simulink model "A03_L5_2"  (R2018b)
settings: Solver=ode45  StartTime=0.0  StopTime=60  MaxStep=0.01  RelTol=1e-3  EnableMultiTasking=on
values from neighbouring files (symbols this model uses):
  K = 2    [A04_L5_script.m]
  T = 1.1+0.3*a+0.6*b    (= 3.5)    [A04_L5_script.m]
  y0 = 0    [A04_L5_script.m]
settings Model: Creator=User  LastModifiedBy=DRAGOMIR
settings DataIOCC: LimitDataPoints=on  SaveFormat=Array
settings OptimizationCC: LifeSpan=inf
settings DebuggingCC: SolverPrmCheckMsg=warning  SFUnexpectedBacktrackingDiag=warning  SFNoUnconditionalDefaultTransitionDiag=warning  SFExecutionAtInitializationDiag=none
settings HardwareCC: ProdBitPerPointer=32  ProdBitPerSizeT=32  ProdBitPerPtrDiffT=32  ProdLargestAtomicFloat=None  ProdIntDivRoundTo=Undefined  ProdEndianess=Unspecified  ProdWordSize=32  ProdHWDeviceType=32-bit Generic
settings ModelReferenceCC: PropagateSignalLabelsOutOfModel=off
settings SFSimCC: SimUseLocalCustomCode=off
settings RTWCC: RTWUseLocalCustomCode=off
settings CodeAppCC: StateflowObjectComments=on
settings GRTTargetCC: TargetLangStandard=C89/C90 (ANSI)  GeneratePreprocessorConditionals=Disable all
settings ConfigComp: CovMetricSettings=dw  CovHtmlReporting=on  CovSaveCumulativeToWorkspaceVar=on  CovSaveSingleToWorkspaceVar=on  CovExternalEMLEnable=off  CovSFcnEnable=off

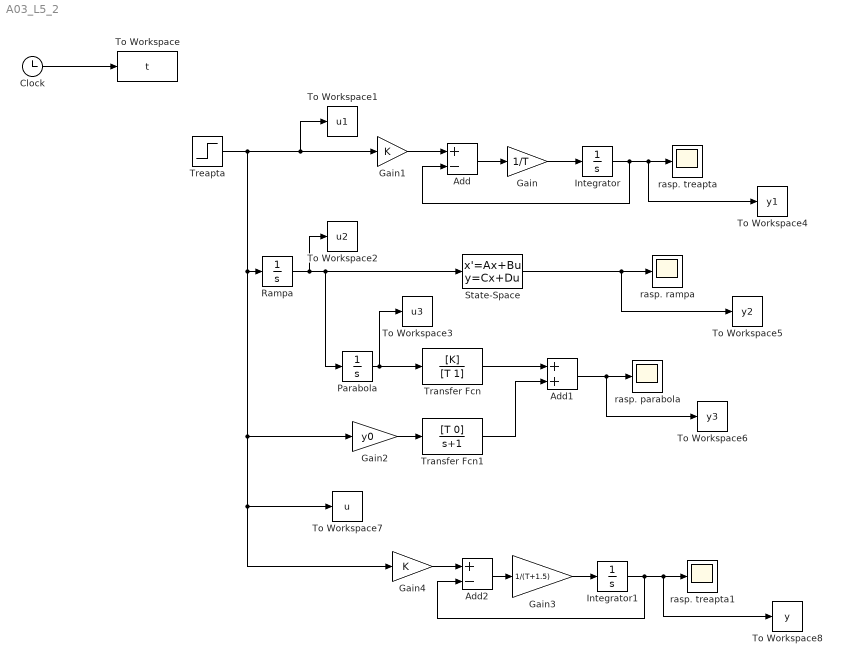
== system A03_L5_2 ==
  Add : Sum  Inputs=+-
  Add1 : Sum
  Add2 : Sum  Inputs=+-
  Clock : Clock
  Gain : Gain  Gain=1/T
  Gain1 : Gain  Gain=K
  Gain2 : Gain  Gain=y0
  Gain3 : Gain  Gain=1/(T+1.5)
  Gain4 : Gain  Gain=K
  Integrator : Integrator  InitialCondition=y0
  Integrator1 : Integrator  InitialCondition=y0
  Parabola : Integrator
  Rampa : Integrator
  State-Space : StateSpace  A=-1/T  B=K/T  D=0  InitialCondition=y0
  To Workspace : ToWorkspace  VariableName=t  SampleTime=-1
  To Workspace1 : ToWorkspace  VariableName=u1  SampleTime=-1
  To Workspace2 : ToWorkspace  VariableName=u2  SampleTime=-1
  To Workspace3 : ToWorkspace  VariableName=u3  SampleTime=-1
  To Workspace4 : ToWorkspace  VariableName=y1  SampleTime=-1
  To Workspace5 : ToWorkspace  VariableName=y2  SampleTime=-1
  To Workspace6 : ToWorkspace  VariableName=y3  SampleTime=-1
  To Workspace7 : ToWorkspace  VariableName=u  SampleTime=-1
  To Workspace8 : ToWorkspace  VariableName=y  SampleTime=-1
  Transfer Fcn : TransferFcn  Numerator=[K]  Denominator=[T 1]
  Transfer Fcn1 : TransferFcn  Numerator=[T 0]  Denominator=[1 1]
  Treapta : Step  Time=0  SampleTime=0
  rasp. parabola : Scope
  rasp. rampa : Scope
  rasp. treapta : Scope
  rasp. treapta1 : Scope
  wires:
  Clock/1 -> To Workspace/1
  Gain/1 -> Integrator/1
  Add/1 -> Gain/1
  Gain1/1 -> Add/1
  Integrator/1 -> To Workspace4/1, rasp. treapta/1, Add/2
  State-Space/1 -> To Workspace5/1, rasp. rampa/1
  Parabola/1 -> Transfer Fcn/1, To Workspace3/1
  Gain2/1 -> Transfer Fcn1/1
  Transfer Fcn/1 -> Add1/1
  Transfer Fcn1/1 -> Add1/2
  Add1/1 -> To Workspace6/1, rasp. parabola/1
  Rampa/1 -> To Workspace2/1, Parabola/1, State-Space/1
  Treapta/1 -> To Workspace7/1, Gain4/1, Gain2/1, Rampa/1, To Workspace1/1, Gain1/1
  Gain3/1 -> Integrator1/1
  Add2/1 -> Gain3/1
  Gain4/1 -> Add2/1
  Integrator1/1 -> To Workspace8/1, rasp. treapta1/1, Add2/2
